simulink library "Resident_Task44"  (R2018b)
settings: Solver=ode45  StartTime=0.0  StopTime=10.0  RelTol=1e-3  EnableMultiTasking=on
libraries: carnot x4
settings Model: Creator=lena.frank  LastModifiedBy=drhf
settings DataIOCC: LimitDataPoints=on  SaveFormat=Array  SignalLoggingSaveFormat=ModelDataLogs
settings OptimizationCC: ExpressionDepthLimit=2147483647  LifeSpan=inf
settings DebuggingCC: UnderspecifiedInitializationDetection=Classic  MergeDetectMultiDrivingBlocksExec=none  SolverPrmCheckMsg=warning  FcnCallInpInsideContextMsg=warning  StateNameClashWarn=warning  SFUnexpectedBacktrackingDiag=warning  SFNoUnconditionalDefaultTransitionDiag=warning  SFExecutionAtInitializationDiag=none
settings HardwareCC: ProdBitPerPointer=32  ProdBitPerSizeT=32  ProdBitPerPtrDiffT=32  ProdLargestAtomicFloat=None  ProdIntDivRoundTo=Undefined  ProdEndianess=Unspecified  ProdWordSize=32  ProdHWDeviceType=32-bit Generic
settings ModelReferenceCC: PropagateSignalLabelsOutOfModel=off
settings SFSimCC: SimUseLocalCustomCode=off
settings RTWCC: RTWUseLocalCustomCode=off
settings CodeAppCC: StateflowObjectComments=on
settings GRTTargetCC: TargetLangStandard=C89/C90 (ANSI)  GeneratePreprocessorConditionals=Disable all  CombineOutputUpdateFcns=off  GRTInterface=on
settings ConfigComp: CovMetricSettings=dw  CovHtmlReporting=on  CovSaveCumulativeToWorkspaceVar=on  CovSaveSingleToWorkspaceVar=on  CovExternalEMLEnable=off

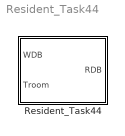
== system Resident_Task44 ==
  Resident_Task44 : Subsystem  mask(Resident Task){period=24*3600, rep_seq_te=[0 1 6 7 8 9 11 12 13 18 19 20 22 23]*3600, rep_seq_de=[1 5 1 1 1 2 1 1 4 2 1 2 1 1]*3600, rep_seq_ye=[105 55 392.5 457.5 420 55 250 55 120 170 615 420 442.5 355], rep_seq_to=[0 6 7 8 9 11 12 13 14 15 17 18 20 21 22]*3600, rep_seq_do=[6 1 1 1 2 1 1 1 1 2 1 2 1 1 2]*3600, rep_seq_yo=[4 2 3 2 0 1 3 2 1 0 1 2 4 3 4]*60, Topen=24, Tclose=23, TrAboveTa=2, TaTooCold=12, timeFIR=24, TaIni=12, starttime=8, stoptime=22, TroomShadeOn=23.8, TroomShadeOff=22.8, SolarShadeOn=300, SolarShadeOff=200, max_shade=1, CalcAirComp=off, mdotCO2=0, mdotH2O=0, mdotVOC=0}
      mask prompts: period "Time period in s"; rep_seq_te "Time values in s"; rep_seq_de "Duration in s"; rep_seq_ye "Internal gains due to electricity consumption in W"; rep_seq_to "Time values in s"; rep_seq_do "Duration in s"; rep_seq_yo "Internal gain due to persons in W"; Topen "Open window if Troom is above [°C]"; Tclose "Close window if Troom is below [°C]"; TrAboveTa "Open window if Troom is above Tamb [K]"; TaTooCold "Close window if average Tamb is below [°C]"; timeFIR "Average time for Tamb in h (only integer values)"; TaIni "Initial value for Tamb in °C"; starttime "Start time in the morning [h]"; stoptime "Stop time in the evening [h]"; TroomShadeOn "Room temperature to switch shading on in °C"; TroomShadeOff "Room temperature to switch shading off in °C"; SolarShadeOn "Solar radiation to switch shading on in W/m²"; SolarShadeOff "Solar radiation to switch shading off in W/m²"; max_shade "Maximum value for Sunshade"; CalcAirComp "Calculate the composition of room air (H2O, CO2, VOC)"; mdotCO2 "Massflow CO2 in kg/s"; mdotH2O "Massflow H2O in kg/s"; mdotVOC "Massflow VOC in kg/s"
      mask help: Create the Resident Data Bus for boundary conditions of Task 44.
      mask TypeOptions period: Electric_Gains_Profile/period | Occupation_Profile/period
      mask TypeOptions rep_seq_te: Electric_Gains_Profile/rep_seq_t
      mask TypeOptions rep_seq_de: Electric_Gains_Profile/rep_seq_d
      mask TypeOptions rep_seq_ye: Electric_Gains_Profile/rep_seq_y
      mask TypeOptions rep_seq_to: Occupation_Profile/rep_seq_t
      mask TypeOptions rep_seq_do: Occupation_Profile/rep_seq_d
      mask TypeOptions rep_seq_yo: Occupation_Profile/rep_seq_y
      mask TypeOptions Topen: Window_Control/Topen
      mask TypeOptions Tclose: Window_Control/Tclose
      mask TypeOptions TrAboveTa: Window_Control/TrAboveTa
      mask TypeOptions TaTooCold: Window_Control/TaTooCold
      mask TypeOptions timeFIR: Window_Control/timeFIR
      mask TypeOptions TaIni: Window_Control/TaIni
      mask TypeOptions starttime: Window_Control/starttime
      mask TypeOptions stoptime: Window_Control/stoptime
      mask TypeOptions TroomShadeOn: Shading_Control/TroomShadeOn
      mask TypeOptions TroomShadeOff: Shading_Control/TroomShadeOff
      mask TypeOptions SolarShadeOn: Shading_Control/SolarShadeOn
      mask TypeOptions SolarShadeOff: Shading_Control/SolarShadeOff
      mask TypeOptions max_shade: Shading_Control/max_shade
      mask TypeOptions CalcAirComp: CalculateAirComposition/CalcAirComp
      mask TypeOptions mdotCO2: Massflow_CO2/Value
      mask TypeOptions mdotH2O: Massflow_H2O/Value
      mask TypeOptions mdotVOC: Massflow_VOC/Value
      mask DialogControl Container5 Prompt: Internal gain
      mask DialogControl Container6 Prompt: Electric gains profile
      mask DialogControl Container7 Prompt: Occupation profile
      mask DialogControl Container8 Prompt: Windows
      mask DialogControl Container10 Prompt: Ventilation cooling
      mask DialogControl Container9 Prompt: Shading
      mask DialogControl Container11 Prompt: Emissions
      mask Display:
      | plot(0,0,100,100,[30,70,70,30,30],[80,80,30,30,80],...
      |     [65,60,40,35],[30,40,40,30],...
      |     [53,53,56,56,50,44,44,47,47],...
      |     [40,45,49,60,65,60,50,45,40],...
      |     [57,50,44],[40,34,40],...
      |     [52,53],[55,55],[47,48],[55,55],...
      |     [56,53,47,44],[51,60,60,51],[52,50,48],[49,48,49])
      | disp('\n\n\n\n\nTASK 44')

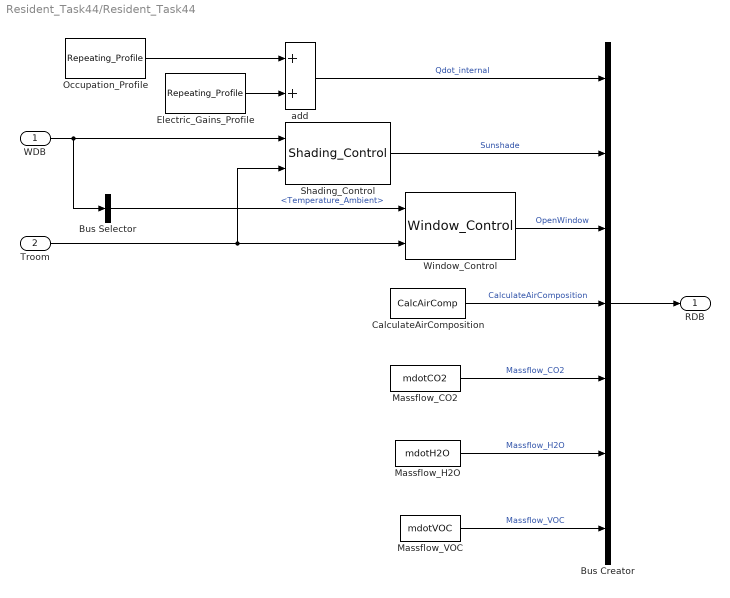
== system Resident_Task44/Resident_Task44 ==
  WDB : Inport
  Troom : Inport  Port=2
  Bus Creator : BusCreator  Inputs=7
  Bus Selector : BusSelector  OutputSignals=Temperature_Ambient
  CalculateAirComposition : Constant  Value=CalcAirComp  mask{CalcAirComp=off}
      mask prompts: CalcAirComp "Calculate the composition of room air (H2O, CO2, VOC)"
  Electric_Gains_Profile : carnot/Load/General/Repeating_Profile  period=period  rep_seq_t=rep_seq_te  rep_seq_d=rep_seq_de  rep_seq_y=rep_seq_ye
      settings: SourceProductName=Carnot
  Massflow_CO2 : Constant  Value=mdotCO2
  Massflow_H2O : Constant  Value=mdotH2O
  Massflow_VOC : Constant  Value=mdotVOC
  Occupation_Profile : carnot/Load/General/Repeating_Profile  period=period  rep_seq_t=rep_seq_to  rep_seq_d=rep_seq_do  rep_seq_y=rep_seq_yo
      settings: SourceProductName=Carnot
  Shading_Control : carnot/Control/Shading_Control  TroomShadeOn=TroomShadeOn  TroomShadeOff=TroomShadeOff  SolarShadeOn=SolarShadeOn  SolarShadeOff=SolarShadeOff  max_shade=max_shade
      settings: SourceProductName=Carnot
  Window_Control : carnot/Control/Window_Control  Topen=Topen  Tclose=Tclose  TrAboveTa=TrAboveTa  TaTooCold=TaTooCold  timeFIR=timeFIR  TaIni=TaIni  starttime=starttime  stoptime=stoptime
      settings: SourceProductName=Carnot
  add : Sum  Inputs=2
  RDB : Outport
  wires:
  WDB/1 -> Shading_Control/1, Bus Selector/1
  Troom/1 -> Shading_Control/2, Window_Control/2
  Bus Selector/1 -> Window_Control/1  "<Temperature_Ambient>"
  Shading_Control/1 -> Bus Creator/2  "Sunshade"
  Bus Creator/1 -> RDB/1
  Window_Control/1 -> Bus Creator/3  "OpenWindow"
  add/1 -> Bus Creator/1  "Qdot_internal"
  Electric_Gains_Profile/1 -> add/2
  Occupation_Profile/1 -> add/1
  Massflow_CO2/1 -> Bus Creator/5  "Massflow_CO2"
  Massflow_H2O/1 -> Bus Creator/6  "Massflow_H2O"
  Massflow_VOC/1 -> Bus Creator/7  "Massflow_VOC"
  CalculateAirComposition/1 -> Bus Creator/4  "CalculateAirComposition"
